simulink model "AUVdepthHeadingControlWithRealisticWind"  (R2024b)
settings: Solver=ode4  StartTime=0.0  StopTime=3600  FixedStep=0.05  RelTol=1e-3  EnableMultiTasking=on
model workspace (MAT data in the model file):
  tau_val = 20
undefined symbols (not defined in the file or in its folder): active_seed, CourseControlToggle, Final_depth, Final_heading, Initial_depth, Initial_heading, Kdz, Kiz, Kpz, WindConditionsEnum
libraries: simulink x3, mssSimulink x3, simulink_extras x1
settings Model: Creator=thor  LastModifiedBy=16178
settings SolverCC: AlgebraicLoopSolver=TrustRegion
settings DataIOCC: SignalLoggingSaveFormat=ModelDataLogs  ReturnWorkspaceOutputs=off
settings OptimizationCC: BooleanDataType=off  InitFltsAndDblsToZero=on  LifeSpan=inf
settings DebuggingCC: SaveWithParameterizedLinksMsg=none  UnderspecifiedInitializationDetection=Classic  MergeDetectMultiDrivingBlocksExec=none  SignalResolutionControl=TryResolveAllWithWarning  MultiTaskDSMMsg=warning  MultiTaskCondExecSysMsg=none  FcnCallInpInsideContextMsg=warning  UnconnectedInputMsg=warning  UnconnectedOutputMsg=warning  UnconnectedLineMsg=warning  SFUnexpectedBacktrackingDiag=warning  SFNoUnconditionalDefaultTransitionDiag=warning  SFExecutionAtInitializationDiag=none  ArithmeticOperatorsInVariantConditions=warning
settings HardwareCC: ProdBitPerPointer=32  ProdBitPerSizeT=32  ProdBitPerPtrDiffT=32  ProdLargestAtomicFloat=None  ProdIntDivRoundTo=Undefined  ProdEndianess=Unspecified  ProdWordSize=32  ProdHWDeviceType=32-bit Generic  TargetUnknown=on
settings ModelReferenceCC: EnableRefExpFcnMdlSchedulingChecks=on  PropagateSignalLabelsOutOfModel=off
settings RTWCC: GPUComputeCapability=3.5  DLArmComputeVersion=19.05
settings CodeAppCC: StateflowObjectComments=on
settings GRTTargetCC: TargetFcnLib=ansi_tfl_tmw.mat  TargetLangStandard=C89/C90 (ANSI)  ModelReferenceCompliant=off  CombineOutputUpdateFcns=off  MatFileLogging=off  GRTInterface=on
settings ConfigComp: CovMetricSettings=dw  CovSaveCumulativeToWorkspaceVar=on  CovSaveSingleToWorkspaceVar=on

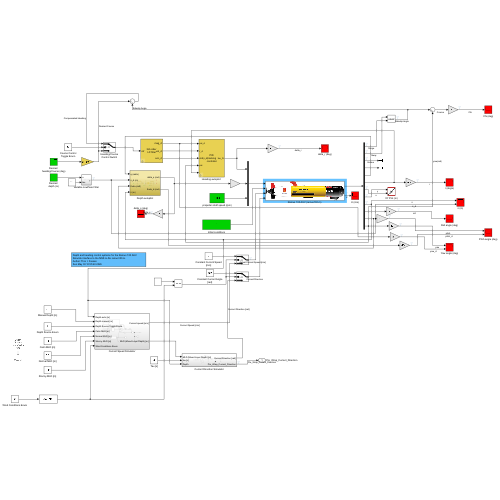
[thumbnail: Simulink's stored preview of the top-level diagram]
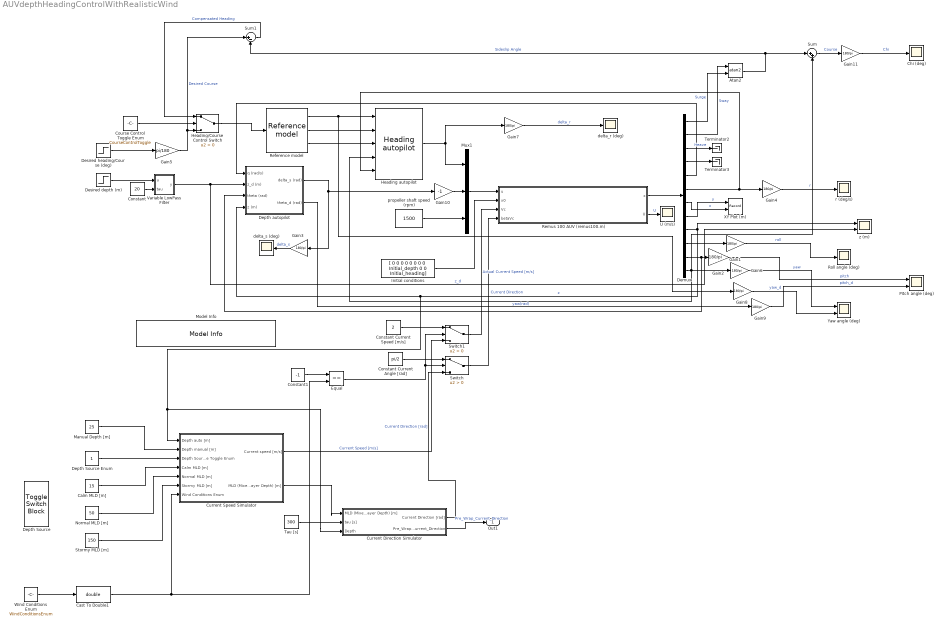
== system AUVdepthHeadingControlWithRealisticWind ==
  Atan2 : Trigonometry  Operator=atan2
  Calm MLD [m] : Constant  Value=15
  Cast To Double1 : DataTypeConversion  OutDataTypeStr=double  SaturateOnIntegerOverflow=off  RndMeth=Floor
  Chi (deg) : Scope
  Constant : Constant  Value=20
  Constant Current Angle [rad] : Constant  Value=pi/2
  Constant Current Speed [m/s] : Constant  Value=2
  Constant1 : Constant  Value=-1
  Course Control Toggle Enum : Constant  Value=CourseControlToggle
  Current Direction Simulator : Subsystem
  Current Speed Simulator : Subsystem
  Demux : Demux  Outputs=12
  Depth Source : ToggleSwitchBlock
      settings: Values={{'Manual', 'Auto'}, [0 1]}
  Depth Source Enum : Constant
  Depth autopilot : Subsystem
  Desired depth (m) : Step  Time=0  Before=Initial_depth  After=Final_depth  SampleTime=0.05
  Desired heading/Course (deg) : Step  Time=0  Before=Initial_heading  After=Final_heading  SampleTime=0
  Equal : RelationalOperator  Operator===  OutDataTypeStr=boolean  RndMeth=Simplest  InputSameDT=off
  Gain{1..4,6..9,11} (9 alike) : Gain  Gain=180/pi
  Gain10 : Gain  Gain=-1
  Gain5 : Gain  Gain=pi/180
  "Heading autopilot " : mssSimulink/Control/Autopilots/Heading autopilot  T_nomoto=5  K_nomoto=1  Kp=1.875  Td=5.333  Ti=20
  Heading/Course Control Switch : Switch  Criteria=u2 > Threshold  SaturateOnIntegerOverflow=off  InputSameDT=off
  Initial conditions : Constant  Value="[ 0 0 0 0 0 0 0 0  Initial_depth 0 0 Initial_heading]"
  Manual Depth [m] : Constant  Value=25
  Model Info : simulink/Model-Wide Utilities/Model Info  Frame=on  DisplayStringWithTags=|  HorizontalTextAlignment=Left  LeftAlignmentValue=0.02
      | Depth and heading control systems for the Remus 100 AUV.
      | Simulink interface to the MSS m-file remus100.m.
      | Author: Thor I. Fossen
      | %<LastModificationDate>
  Mux1 : Mux  Inputs=3
  Normal MLD [m] : Constant  Value=50
  Pitch angle (deg) : Scope  NumInputPorts=2
  Reference model : mssSimulink/Guidance/Reference model  v_max=10  zeta_d=1.0  w_d=0.2
  "Remus 100 AUV (remus100.m) " : Subsystem  AncestorBlock=mssSimulink/Marine craft models/Remus 100 AUV (remus100.m)
      mask Display: image('remus100.jpg'); % Use "Edit Image" on toolstrip to change.
  Roll angle (deg) : Scope
  Stormy MLD [m] : Constant  Value=150
  Sum : Sum  Inputs=|++
  Sum1 : Sum  Inputs=|+-
  Switch : Switch  Criteria=u2 > Threshold  SaturateOnIntegerOverflow=off  InputSameDT=off
  Switch1 : Switch  Criteria=u2 > Threshold  SaturateOnIntegerOverflow=off  InputSameDT=off
  Tau [s] : Constant  Value=300
  Terminator2 : Terminator
  Terminator3 : Terminator
  U (m/s) : Scope
  Variable LowPass Filter : Subsystem
  Wind Conditions Enum : Constant  Value=WindConditionsEnum
  XY Plot (m) : Record  FileSettingsInternal="{\"entries\":[{\"content\":{\"excelSettings\":{\"content\":{},\"type\":\"Streamout.ExcelSettings\"}},\"type\":\"Streamout.FileSettingStorage\",\"uuid\":\"\"}],\"packageUris\":[\"http:\\/\\/schema.mathworks.com\\/mf0\\/streamout_blocks\\/R2020a\"],\"version\":\"1.0\"}"  Layout=[1 1]  SignalsInternal="{\"entries\":[{\"content\":{\"signals\":[{\"content\":{\"blockPath\":[],\"dimensions\":[1],\"domain\":\"\",\"lineColor\":\"#b746ff\",\"lineWidth\":2,\"port\":1,\"sid\":[\"\"],\"signalID\":1,\"signalName\":\"y\"},\"type\":\"RecordBlkView.Signal\",\"uuid\":\"\"},{\"content\":{\"blockPath\":[],\"dimensions\":[1],\"domain\":\"\",\"lineColor\":\"#64d413\",\"lineWidth\":2,\"port\":2,\"sid\":[\"\"],\"signalID\":2,\"signalName\":\"x\"},\"type\":\"RecordBlkView.Signal\",\"uuid\":\"\"}]},\"type\":\"RecordBlkView.InputSignals\",\"uuid\":\"\"}],\"packageUris\":[\"http:\\/\\/schema.mathworks.com\\/mf0\\/streamout_blocks\\/R2020a\"],\"version\":\"1.0\"}"  VisualizationBindings="{\"xyplotplugin\":{\"info\":[{\"series\":[],\"subplotID\":1}]}}"  CompatibilityTag=XY  st=-1
  Yaw angle (deg) : Scope  NumInputPorts=2
  delta_r (deg) : Scope
  delta_s (deg) : Scope
  propeller shaft speed (rpm) : Constant  Value=1500
  r (deg/s) : Scope
  z (m) : Scope  NumInputPorts=2
  Out1 : Outport  SignalName=Pre_Wrap_Current_Direction
  wires:
  Initial conditions/1 -> "Remus 100 AUV (remus100.m) "/2(x0)
  Mux1/1 -> "Remus 100 AUV (remus100.m) "/1(u)
  "Heading autopilot "/1 -> Gain7/1, Mux1/1
  propeller shaft speed (rpm)/1 -> Mux1/3
  Demux/2 -> Atan2/1  "Sway"
  Gain1/1 -> Roll angle (deg)/1  "roll"
  Demux/7 -> XY Plot (m)/2  "x"
  "Remus 100 AUV (remus100.m) "/1(x) -> Demux/1
  Demux/4 -> Terminator3/1
  "Remus 100 AUV (remus100.m) "/2(U) -> U (m/s)/1  "U"
  Demux/5 -> Depth autopilot/1(q (rad/s))
  Demux/1 -> Atan2/2  "Surge"
  Demux/10 -> Gain1/1
  Gain6/1 -> Yaw angle (deg)/1  "yaw"
  Gain4/1 -> r (deg/s)/1  "r"
  Gain2/1 -> Pitch angle (deg)/1  "pitch"
  Demux/8 -> XY Plot (m)/1  "y"
  Demux/6 -> "Heading autopilot "/5, Gain4/1
  Demux/12 -> "Heading autopilot "/4, Sum/2, Gain6/1  "yaw(rad)"
  Demux/9 -> z (m)/1, Current Direction Simulator/3(Depth), Current Speed Simulator/1(Depth auto [m]), Depth autopilot/4(z (m))  "z"
  Depth autopilot/1(delta_s (rad)) -> Gain3/1, Gain10/1
  Desired depth (m)/1 -> Variable LowPass Filter/1(u)
  Demux/11 -> Gain2/1, Depth autopilot/3(theta (rad))
  Gain3/1 -> delta_s (deg)/1  "delta_s"
  Desired heading/Course (deg)/1 -> Gain5/1
  Reference model/1 -> Gain8/1, "Heading autopilot "/1
  Reference model/2 -> "Heading autopilot "/2
  Reference model/3 -> "Heading autopilot "/3
  Gain7/1 -> delta_r (deg)/1  "delta_r"
  Demux/3 -> Terminator2/1  "Heave"
  Current Direction Simulator/1(Current Direction [rad]) -> Switch/3  "Current Direction [rad]"
  Gain8/1 -> Yaw angle (deg)/2  "yaw_d"
  Variable LowPass Filter/1(y) -> z (m)/2, Depth autopilot/2(z_d (m))  "z_d"
  Depth autopilot/2(theta_d (rad)) -> Gain9/1
  Gain9/1 -> Pitch angle (deg)/2  "pitch_d"
  Gain10/1 -> Mux1/2
  Manual Depth [m]/1 -> Current Speed Simulator/2(Depth manual [m])
  Depth Source Enum/1 -> Current Speed Simulator/3(Depth Source Toggle Enum)
  Calm MLD [m]/1 -> Current Speed Simulator/4(Calm MLD [m])
  Normal MLD [m]/1 -> Current Speed Simulator/5(Normal MLD [m])
  Stormy MLD [m]/1 -> Current Speed Simulator/6(Stormy MLD [m])
  Wind Conditions Enum/1 -> Cast To Double1/1
  Current Speed Simulator/1(Current speed [m/s]) -> Switch1/3  "Current Speed [m/s]"
  Current Speed Simulator/2(MLD (Mixed Layer Depth) [m]) -> Current Direction Simulator/1(MLD (Mixed Layer Depth) [m])
  Tau [s]/1 -> Current Direction Simulator/2(tau [s])
  Current Direction Simulator/2(Pre_Wrap_Current_Direction) -> Out1/1  "Pre_Wrap_Current_Direction"
  Constant/1 -> Variable LowPass Filter/2(tau)
  Atan2/1 -> Sum/1, Sum1/2  "Sideslip Angle"
  Sum/1 -> Gain11/1  "Course"
  Gain5/1 -> Sum1/1, Heading/Course Control Switch/3  "Desired Course"
  Heading/Course Control Switch/1 -> Reference model/1
  Sum1/1 -> Heading/Course Control Switch/1  "Compensated Heading"
  Gain11/1 -> Chi (deg)/1  "Chi"
  Course Control Toggle Enum/1 -> Heading/Course Control Switch/2
  Equal/1 -> Switch/2, Switch1/2
  Constant1/1 -> Equal/1
  Constant Current Angle [rad]/1 -> Switch/1
  Constant Current Speed [m/s]/1 -> Switch1/1
  Switch1/1 -> "Remus 100 AUV (remus100.m) "/3(Vc)  "Actual Current Speed [m/s]"
  Switch/1 -> "Remus 100 AUV (remus100.m) "/4(betaVc)  "Current Direction"
  Cast To Double1/1 -> Equal/2, Current Speed Simulator/7(Wind Conditions Enum)

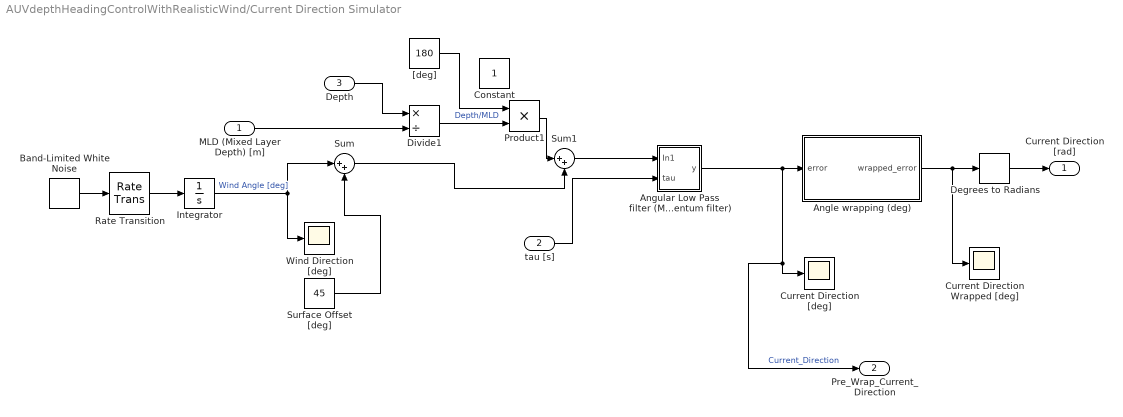
== system AUVdepthHeadingControlWithRealisticWind/Current Direction Simulator ==
  MLD (Mixed Layer Depth) [m] : Inport
  tau [s] : Inport  Port=2
  Depth : Inport  Port=3
  Angle wrapping (deg) : MATLAB Function  TreatAsAtomicUnit=on
  Angular Low Pass filter (Momentum filter) : Subsystem
  Band-Limited White Noise : simulink/Sources/Band-Limited White Noise  Cov=[0.1]  Ts=0.1  seed=active_seed+1
  Constant : Constant
  Current Direction Wrapped [deg] : Scope
  Current Direction [deg] : Scope
  Degrees to Radians : simulink_extras/Transformations/Degrees to Radians
  Divide1 : Product  Inputs=*/
  Integrator : Integrator
  Product1 : Product
  Rate Transition : RateTransition
  Sum : Sum  Inputs=|++
  Sum1 : Sum  Inputs=|++
  Surface Offset [deg] : Constant  Value=45
  Wind Direction [deg] : Scope
  "[deg]" : Constant  Value=180
  Current Direction [rad] : Outport
  Pre_Wrap_Current_Direction : Outport  Port=2
  wires:
  Angle wrapping (deg)/1(wrapped_error) -> Current Direction Wrapped [deg]/1, Degrees to Radians/1
  Surface Offset [deg]/1 -> Sum/2
  Divide1/1 -> Product1/2  "Depth/MLD"
  Band-Limited White Noise/1 -> Rate Transition/1
  Integrator/1 -> Sum/1, Wind Direction [deg]/1  "Wind Angle [deg]"
  Sum/1 -> Sum1/2
  Angular Low Pass filter (Momentum filter)/1(y) -> Pre_Wrap_Current_Direction/1, Current Direction [deg]/1, Angle wrapping (deg)/1(error)  "Current_Direction"
  Sum1/1 -> Angular Low Pass filter (Momentum filter)/1(In1)
  Rate Transition/1 -> Integrator/1
  tau [s]/1 -> Angular Low Pass filter (Momentum filter)/2(tau)
  Degrees to Radians/1 -> Current Direction [rad]/1
  MLD (Mixed Layer Depth) [m]/1 -> Divide1/2
  Product1/1 -> Sum1/1
  "[deg]"/1 -> Product1/1
  Depth/1 -> Divide1/1

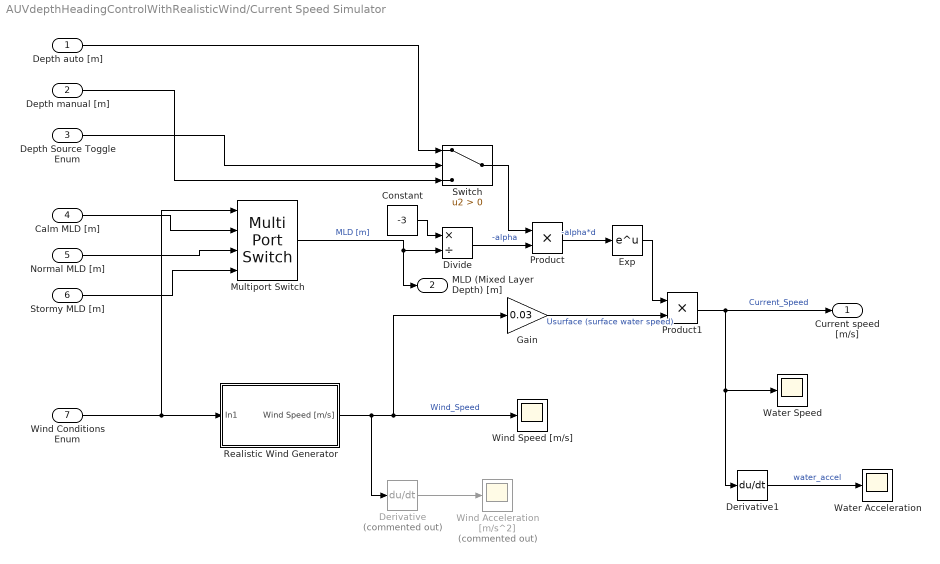
== system AUVdepthHeadingControlWithRealisticWind/Current Speed Simulator ==
  Depth auto [m] : Inport
  Depth manual [m] : Inport  Port=2
  Depth Source Toggle Enum : Inport  Port=3
  Calm MLD [m] : Inport  Port=4
  Normal MLD [m] : Inport  Port=5
  Stormy MLD [m] : Inport  Port=6
  Wind Conditions Enum : Inport  Port=7
  Constant : Constant  Value=-3
  Derivative : Derivative  Commented=on
  Derivative1 : Derivative
  Divide : Product  Inputs=*/
  Exp : Math
  Gain : Gain  Gain=0.03
  Multiport Switch : MultiPortSwitch  DataPortOrder=Specify indices  DiagnosticForDefault=Warning  SaturateOnIntegerOverflow=off  InputSameDT=off
  Product : Product
  Product1 : Product
  Realistic Wind Generator : Subsystem
  Switch : Switch  Criteria=u2 > Threshold  SaturateOnIntegerOverflow=off  InputSameDT=off
  Water Acceleration : Scope
  Water Speed : Scope
  Wind Acceleration [m/s^2] : Scope  Commented=on
  Wind Speed [m/s] : Scope
  Current speed [m/s] : Outport
  MLD (Mixed Layer Depth) [m] : Outport  Port=2
  wires:
  Derivative/1 -> Wind Acceleration [m/s^2]/1
  Exp/1 -> Product1/1
  Realistic Wind Generator/1(Wind Speed [m/s]) -> Derivative/1, Gain/1, Wind Speed [m/s]/1  "Wind_Speed"
  Product/1 -> Exp/1  "-alpha*d"
  Switch/1 -> Product/1
  Depth Source Toggle Enum/1 -> Switch/2
  Product1/1 -> Current speed [m/s]/1, Water Speed/1, Derivative1/1  "Current_Speed"
  Derivative1/1 -> Water Acceleration/1  "water_accel"
  Wind Conditions Enum/1 -> Multiport Switch/1, Realistic Wind Generator/1(In1)
  Depth manual [m]/1 -> Switch/3
  Depth auto [m]/1 -> Switch/1
  Multiport Switch/1 -> Divide/2, MLD (Mixed Layer Depth) [m]/1  "MLD [m]"
  Divide/1 -> Product/2  "-alpha"
  Calm MLD [m]/1 -> Multiport Switch/2
  Stormy MLD [m]/1 -> Multiport Switch/4
  Gain/1 -> Product1/2  "Usurface (surface water speed)"
  Constant/1 -> Divide/1
  Normal MLD [m]/1 -> Multiport Switch/3

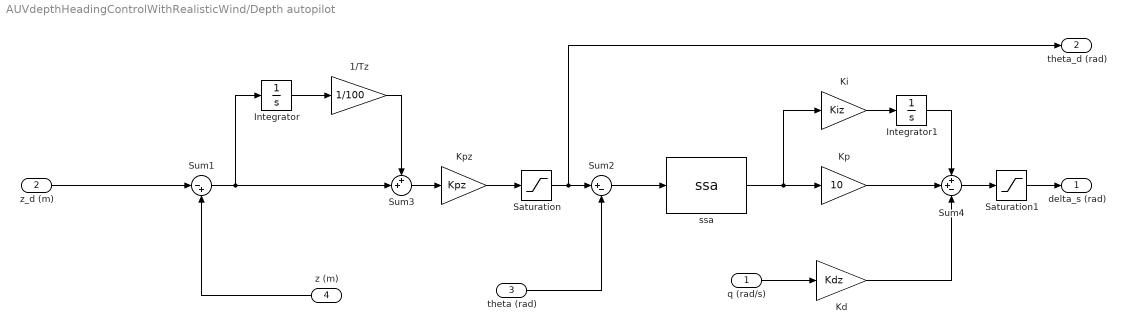
== system AUVdepthHeadingControlWithRealisticWind/Depth autopilot ==
  q (rad/s) : Inport
  z_d (m) : Inport  Port=2
  theta (rad) : Inport  Port=3
  z (m) : Inport  Port=4
  1/Tz : Gain  Gain=1/100  SaturateOnIntegerOverflow=on  OutDataTypeStr=Inherit: Same as input  ParamDataTypeStr=Inherit: Same as input
  Integrator : Integrator
  Integrator1 : Integrator
  Kd : Gain  Gain=Kdz  SaturateOnIntegerOverflow=on  OutDataTypeStr=Inherit: Same as input  ParamDataTypeStr=Inherit: Same as input
  Ki : Gain  Gain=Kiz  SaturateOnIntegerOverflow=on  OutDataTypeStr=Inherit: Same as input  ParamDataTypeStr=Inherit: Same as input
  Kp : Gain  Gain=10  SaturateOnIntegerOverflow=on  OutDataTypeStr=Inherit: Same as input  ParamDataTypeStr=Inherit: Same as input
  Kpz : Gain  Gain=Kpz  SaturateOnIntegerOverflow=on  OutDataTypeStr=Inherit: Same as input  ParamDataTypeStr=Inherit: Same as input
  Saturation : Saturate  UpperLimit=1.35  LowerLimit=-1.35
  Saturation1 : Saturate  UpperLimit=0.35  LowerLimit=-0.35
  Sum1 : Sum  Inputs=|-+  InputSameDT=on  SaturateOnIntegerOverflow=on  OutDataTypeStr=Inherit: Same as first input
  Sum2 : Sum  Inputs=|+-  InputSameDT=on  SaturateOnIntegerOverflow=on  OutDataTypeStr=Inherit: Same as first input
  Sum3 : Sum  Inputs=++|  InputSameDT=on  SaturateOnIntegerOverflow=on  OutDataTypeStr=Inherit: Same as first input
  Sum4 : Sum  Inputs=++-  InputSameDT=on  SaturateOnIntegerOverflow=on  OutDataTypeStr=Inherit: Same as first input
  ssa : mssSimulink/Utilities/Math Operations/ssa  SystemSampleTime=-1  VariantActivationTime=update diagram  AllowFlexibleInterface=on  Latency=0  AutoFrameSizeCalculation=off
  delta_s (rad) : Outport
  theta_d (rad) : Outport  Port=2
  wires:
  Kp/1 -> Sum4/2
  q (rad/s)/1 -> Kd/1
  Sum2/1 -> ssa/1
  z_d (m)/1 -> Sum1/1
  z (m)/1 -> Sum1/2
  Sum1/1 -> Sum3/2, Integrator/1
  Sum3/1 -> Kpz/1
  1/Tz/1 -> Sum3/1
  Integrator/1 -> 1/Tz/1
  Ki/1 -> Integrator1/1
  Integrator1/1 -> Sum4/1
  ssa/1 -> Ki/1, Kp/1
  theta (rad)/1 -> Sum2/2
  Kd/1 -> Sum4/3
  Kpz/1 -> Saturation/1
  Saturation/1 -> theta_d (rad)/1, Sum2/1
  Sum4/1 -> Saturation1/1
  Saturation1/1 -> delta_s (rad)/1

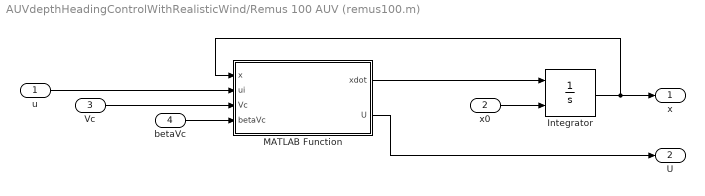
== system AUVdepthHeadingControlWithRealisticWind/Remus 100 AUV (remus100.m)  ==
  u : Inport
  x0 : Inport  Port=2
  Vc : Inport  Port=3
  betaVc : Inport  Port=4
  Integrator : Integrator  InitialConditionSource=external  InitialCondition=[1 1]  UpperSaturationLimit=10  LowerSaturationLimit=-10
  MATLAB Function : MATLAB Function  TreatAsAtomicUnit=on
  x : Outport
  U : Outport  Port=2
  wires:
  Vc/1 -> MATLAB Function/3(Vc)
  betaVc/1 -> MATLAB Function/4(betaVc)
  u/1 -> MATLAB Function/2(ui)
  Integrator/1 -> MATLAB Function/1(x), x/1
  MATLAB Function/1(xdot) -> Integrator/1
  x0/1 -> Integrator/2
  MATLAB Function/2(U) -> U/1

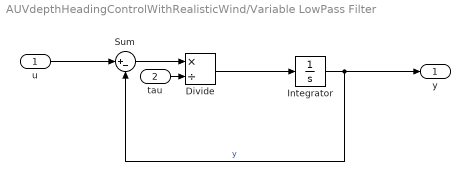
== system AUVdepthHeadingControlWithRealisticWind/Variable LowPass Filter ==
  u : Inport
  tau : Inport  Port=2
  Divide : Product  Inputs=*/
  Integrator : Integrator  InitialCondition=Initial_depth
  Sum : Sum  Inputs=|+-
  y : Outport
  wires:
  u/1 -> Sum/1
  Integrator/1 -> Sum/2, y/1  "y"
  Sum/1 -> Divide/1
  Divide/1 -> Integrator/1
  tau/1 -> Divide/2

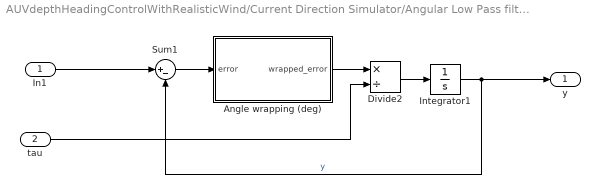
== system AUVdepthHeadingControlWithRealisticWind/Current Direction Simulator/Angular Low Pass filter (Momentum filter) ==
  In1 : Inport
  tau : Inport  Port=2
  Angle wrapping (deg) : MATLAB Function  TreatAsAtomicUnit=on
  Divide2 : Product  Inputs=*/
  Integrator1 : Integrator
  Sum1 : Sum  Inputs=|+-
  y : Outport
  wires:
  tau/1 -> Divide2/2
  Integrator1/1 -> y/1, Sum1/2  "y"
  Divide2/1 -> Integrator1/1
  In1/1 -> Sum1/1
  Angle wrapping (deg)/1(wrapped_error) -> Divide2/1
  Sum1/1 -> Angle wrapping (deg)/1(error)

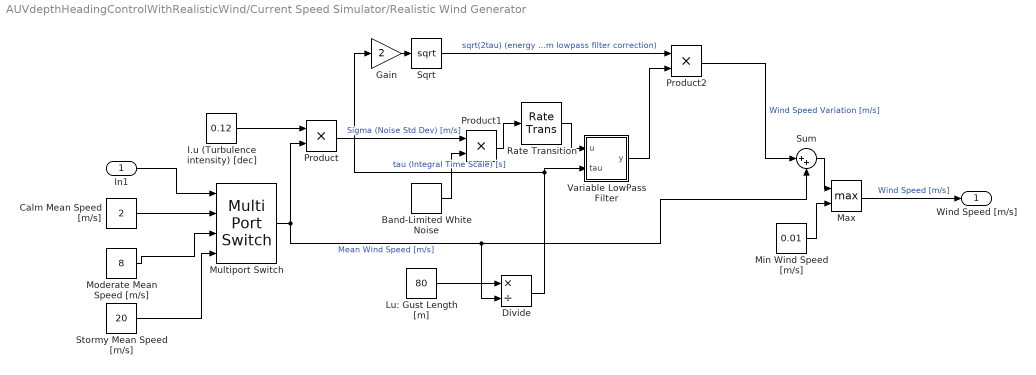
== system AUVdepthHeadingControlWithRealisticWind/Current Speed Simulator/Realistic Wind Generator ==
  In1 : Inport
  Band-Limited White Noise : simulink/Sources/Band-Limited White Noise  Cov=[1]  Ts=0.1  seed=active_seed
  Calm Mean Speed [m/s] : Constant  Value=2
  Divide : Product  Inputs=*/
  Gain : Gain  Gain=2
  I.u (Turbulence intensity) [dec] : Constant  Value=0.12
  Lu: Gust Length [m] : Constant  Value=80
  Max : MinMax  Function=max  Inputs=2
  Min Wind Speed [m/s] : Constant  Value=0.01
  Moderate Mean Speed [m/s] : Constant  Value=8
  Multiport Switch : MultiPortSwitch  DataPortOrder=Specify indices  DiagnosticForDefault=Warning  SaturateOnIntegerOverflow=off  InputSameDT=off
  Product : Product
  Product1 : Product
  Product2 : Product
  Rate Transition : RateTransition
  Sqrt : Sqrt
  Stormy Mean Speed [m/s] : Constant  Value=20
  Sum : Sum  Inputs=|++
  Variable LowPass Filter : Subsystem
  Wind Speed [m/s] : Outport
  wires:
  Max/1 -> Wind Speed [m/s]/1  "Wind Speed [m/s]"
  Sum/1 -> Max/1
  Product/1 -> Product1/1  "Sigma (Noise Std Dev) [m/s]"
  Band-Limited White Noise/1 -> Product1/2
  Min Wind Speed [m/s]/1 -> Max/2
  Stormy Mean Speed [m/s]/1 -> Multiport Switch/4
  Multiport Switch/1 -> Divide/2, Sum/2, Product/2  "Mean Wind Speed [m/s]"
  Moderate Mean Speed [m/s]/1 -> Multiport Switch/3
  I.u (Turbulence intensity) [dec]/1 -> Product/1
  Lu: Gust Length [m]/1 -> Divide/1
  Divide/1 -> Gain/1, Variable LowPass Filter/2(tau)  "tau (Integral Time Scale) [s]"
  Product1/1 -> Rate Transition/1
  Rate Transition/1 -> Variable LowPass Filter/1(u)
  Gain/1 -> Sqrt/1
  Sqrt/1 -> Product2/1  "sqrt(2tau) (energy loss from lowpass filter correction)"
  Variable LowPass Filter/1(y) -> Product2/2
  Product2/1 -> Sum/1  "Wind Speed Variation [m/s]"
  In1/1 -> Multiport Switch/1
  Calm Mean Speed [m/s]/1 -> Multiport Switch/2

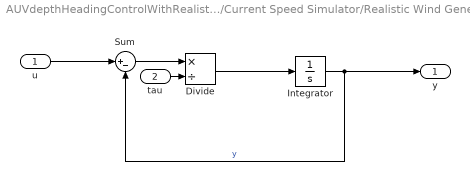
== system AUVdepthHeadingControlWithRealisticWind/Current Speed Simulator/Realistic Wind Generator/Variable LowPass Filter ==
  u : Inport
  tau : Inport  Port=2
  Divide : Product  Inputs=*/
  Integrator : Integrator
  Sum : Sum  Inputs=|+-
  y : Outport
  wires:
  u/1 -> Sum/1
  Integrator/1 -> Sum/2, y/1  "y"
  Sum/1 -> Divide/1
  Divide/1 -> Integrator/1
  tau/1 -> Divide/2

== matlab function AUVdepthHeadingControlWithRealisticWind/Current Direction Simulator/Angle wrapping (deg) ==
  data: error input; wrapped_error output
function wrapped_error = fcn(error)
    wrapped_error = mod(error + 180, 360) - 180;
end

== matlab function AUVdepthHeadingControlWithRealisticWind/Current Direction Simulator/Angular Low Pass filter (Momentum filter)/Angle wrapping (deg) ==
  data: error input; wrapped_error output
function wrapped_error = fcn(error)
    wrapped_error = mod(error + 180, 360) - 180;
end

== matlab function AUVdepthHeadingControlWithRealisticWind/Remus 100 AUV (remus100.m) /MATLAB Function ==
  data: x input; ui input; Vc input; xdot output; U output; betaVc input
function [xdot,U] = fcn(x,ui,Vc,betaVc)
% State vector: x = [ u v w p q r x y z phi theta psi ]' and speed U in m/s  
% (optionally) for the Remus 100 autonomous underwater vehicle (AUV). The 
% length of the AUV is L = 1.7 m, while the state vector is defined as:
%
%  u:       surge velocity          (m/s)
%  v:       sway velocity           (m/s)
%  w:       heave velocity          (m/s)
%  p:       roll rate               (rad/s)
%  q:       pitch rate              (rad/s)
%  r:       yaw rate                (rad/s)
%  x:       North position          (m)
%  y:       East position           (m)
%  z:       downwards position      (m)
%  phi:     roll angle              (rad)
%  theta:   pitch angle             (rad)
%  psi:     yaw angle               (rad)
%
% The control inputs are:
%
%  ui = [ delta_r delta_s n ]'  where
%
%    delta_r:   rudder angle (rad)
%    delta_s:   aft stern plane (rad) 
%    n:         propeller revolution (rpm)
%
% The last arguments Vc and betaVc are optional arguments for ocean current 
% speed and direction expressed in NED. 
    % 1. Explicitly preallocate ALL outputs to lock their memory sizes
    xdot = zeros(12, 1);
    U = 0; % Preallocate the scalar output as well!
    
    % 2. Call the MSS function and catch results in TEMPORARY variables
    [temp_xdot, temp_U] = remus100(x, ui, Vc, betaVc);
    
    % 3. Map the temporary values into your locked-dimension outputs
    % The (:) forces Simulink to preserve the 12x1 shape of xdot
    xdot(:) = temp_xdot;
    U = temp_U;

end
